simulink model "Basics_01"  (R2018a)
settings: Solver=VariableStepAuto  StartTime=0.0  StopTime=Ttot  RelTol=1e-3
values from neighbouring files (symbols this model uses):
  EnableInverter = 1    [Basics_00_Param.m]
  fn = 50    [Basics_00_Param.m]
  idref = 0.0    (= 0)    [Basics_00_Param.m]
  iqref_FinalLevel = -0.2    [Basics_00_Param.m]
  iqref_InitialLevel = 0.0    (= 0)    [Basics_00_Param.m]
  iqref_StepTime = 10000.760    (= 10000.76)    [Basics_00_Param.m]
  Kp = 2    [Basics_00_Param.m]
  L = X / 2 / pi / fn    (= 0.00159154943092)    [Basics_00_Param.m]
  Phi = atan (X/R)    [Basics_00_Param.m]
  R = X/20    (= 0.025)    [Basics_00_Param.m]
  Tau = L / R    (= 0.0636619772368)    [Basics_00_Param.m]
  Ts_control = 1/20000    (= 5e-05)    [Basics_00_Param.m]
  Ts_PWM = 1/200000    (= 5e-06)    [Basics_00_Param.m]
  Udc = Uanp * 3^0.5    (= 1.73205080757)    [Basics_00_Param.m]
  V_NegSeq_FinalValue = 0    [Basics_00_Param.m]
  V_NegSeq_InitialValue = 0.0    (= 0)    [Basics_00_Param.m]
  V_NegSeq_StepTime = 10000.25    [Basics_00_Param.m]
  V_PosSeq_FinalValue = 1    [Basics_00_Param.m]
  V_PosSeq_InitialValue = 1    [Basics_00_Param.m]
  V_PosSeq_StepTime = 10000    [Basics_00_Param.m]
  X = 0.5    [Basics_00_Param.m]
  Z = (X^2 + R^2)^0.5    (= 0.500624609863)    [Basics_00_Param.m]
undefined symbols (not defined in the file or in its folder): DDLPF_Notch, ESS, PCC, Select_AMA
libraries: PhD_Library x18, powerlib x10
settings Model: SimulationMode=accelerator  Creator=daniemot  LastModifiedBy=daniemot
settings SolverCC: AutoInsertRateTranBlk=on
settings DataIOCC: ExternalInput=getinputstruct(WN_50mF_op_snapshot1)  InitialState=getstatestruct(WN_50mF_op_snapshot1)  SaveFinalState=on  SaveFormat=StructureWithTime  SaveOutput=off  SignalLogging=off  DSMLogging=off  SaveTime=off
settings DebuggingCC: ReadBeforeWriteMsg=DisableAll  WriteAfterWriteMsg=DisableAll  WriteAfterReadMsg=DisableAll  MultiTaskDSMMsg=none
settings ModelReferenceCC: UpdateModelReferenceTargets=IfOutOfDate
settings SFSimCC: SFSimEcho=off

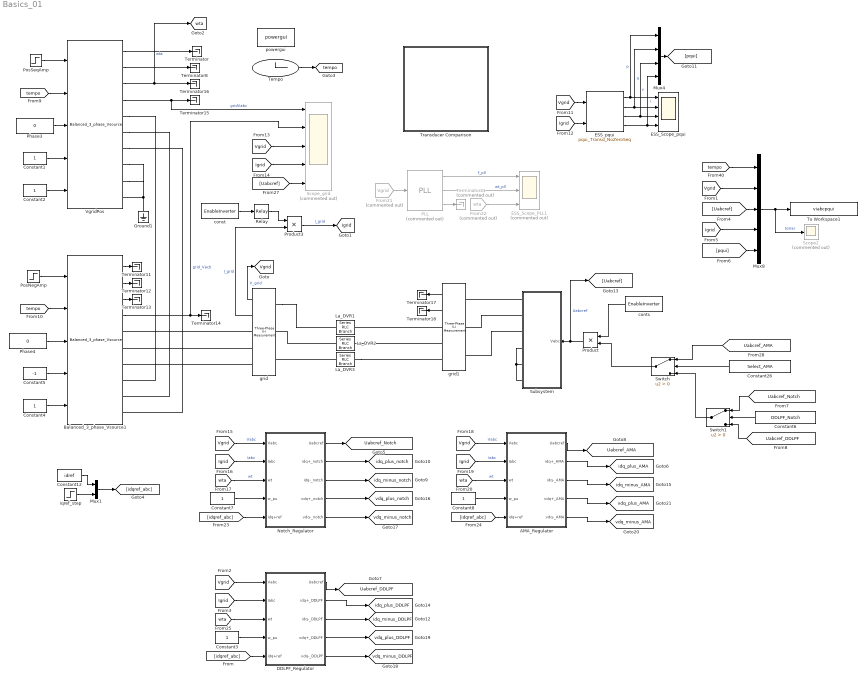
== system Basics_01 ==
  AMA_Regulator : Subsystem
  Balanced_3_phase_Vsource1 : PhD_Library/Offshore_Oil_and_Wind/Balanced_3_phase_Vsource  BaseAmp=Uanp  fn=fn
  Constant{1..4,7..8} (6 alike) : Constant
  Constant12 : Constant  Value=idref
  Constant26 : Constant  Value=Select_AMA
  Constant5 : Constant  Value=-1
  Constant6 : Constant  Value=DDLPF_Notch
  DDLPF_Regulator : Subsystem
  ESS_Scope_PLL1 : Scope  Commented=on  NumInputPorts=3
  ESS_Scope_pqui : Scope  NumInputPorts=4
  ESS_pqui : PhD_Library/Offshore_Oil_and_Wind/pqui_Transd_NoZeroSeq  Sn=3/2  Uanp=1  Iap=1
  From21 : From  Commented=on  GotoTag=Vgrid
  From22 : From  Commented=on  GotoTag=wta
  Ground1 : powerlib/Elements/Ground  LConnTagsString=a
  La_DVR1 : powerlib/Elements/Series RLC Branch  LConnTagsString=__new0  RConnTagsString=__new0  BranchType=RL  Resistance=R  Inductance=L  SetiL0=off  InitialCurrent=0  Capacitance=1.0  Setx0=off  InitialVoltage=0  Measurements=None
  La_DVR2 : powerlib/Elements/Series RLC Branch  LConnTagsString=__new0  RConnTagsString=__new0  BranchType=RL  Resistance=R  Inductance=L  SetiL0=off  InitialCurrent=0  Capacitance=1.0  Setx0=off  InitialVoltage=0  Measurements=None
  La_DVR3 : powerlib/Elements/Series RLC Branch  LConnTagsString=__new0  RConnTagsString=__new0  BranchType=RL  Resistance=R  Inductance=L  SetiL0=off  InitialCurrent=0  Capacitance=1.0  Setx0=off  InitialVoltage=0  Measurements=None
  Mux1 : Mux  Inputs=2
  Mux4 : Mux
  Mux8 : Mux  Inputs=5
  Notch_Regulator : Subsystem
  PLL : PhD_Library/Offshore_Oil_and_Wind/PLL  Commented=on  fn=fn  Ts=Ts_control  Kp_pll=90  Ki_pll=1600  Kd_pll=0  PLL_ini=0
  Phase3 : Constant  Value=0
  Phase4 : Constant  Value=0
  PosNegAmp : Step  Time=V_NegSeq_StepTime  Before=V_NegSeq_InitialValue  After=V_NegSeq_FinalValue
  PosSeqAmp : Step  Time=V_PosSeq_StepTime  Before=V_PosSeq_InitialValue  After=V_PosSeq_FinalValue
  Product : Product
  Product3 : Product
  Relay : Relay  OnSwitchValue=0.5  OffSwitchValue=0.4  OffOutputValue=-1
  Scope2 : Scope  Commented=on
  Scope_grid : Scope  Commented=on  NumInputPorts=5
  Subsystem : Subsystem
  Switch : Switch  Criteria=u2 > Threshold
  Switch1 : Switch  Criteria=u2 > Threshold
  Tempo : Clock
  Terminator{,8,11..18} (10 alike) : Terminator
  Terminator21 : Terminator  Commented=on
  To Workspace1 : ToWorkspace  VariableName=viabcpqui  SampleTime=Ts_control
  Transducer Comparison : Subsystem
  VgridPos : PhD_Library/Offshore_Oil_and_Wind/Balanced_3_phase_Vsource  BaseAmp=Uanp  fn=fn
  const : Constant  Value=EnableInverter
  conts : Constant  Value=EnableInverter
  grid : powerlib/Measurements/Three-Phase V-I Measurement  VoltageMeasurement=phase-to-ground  SetLabelV=off  LabelV=vconv  Vpu=off  VpuLL=off  CurrentMeasurement=yes  SetLabelI=off  LabelI=iconv  Ipu=off  Pbase=sn  Vbase=uab  OutputType=Complex  PhasorSimulation=off  PSBequivalent=0
  grid1 : powerlib/Measurements/Three-Phase V-I Measurement  VoltageMeasurement=phase-to-ground  SetLabelV=off  LabelV=vconv  Vpu=off  VpuLL=off  CurrentMeasurement=yes  SetLabelI=off  LabelI=iconv  Ipu=off  Pbase=sn  Vbase=uab  OutputType=Complex  PhasorSimulation=off  PSBequivalent=0
  iqref_step : Step  Time=iqref_StepTime  Before=iqref_InitialLevel  After=iqref_FinalLevel
  powergui : powerlib/powergui  Priority=1  SimulationMode=Discrete  SampleTime=5e-6  frequency=60  Iterations=50  frequencyindice=0  Pbase=100e6  ErrMax=1e-4  UnitsV=kV  UnitsW=MW  buscounter=0  FunctionMessages=off  echomessages=off  EnableUseOfTLC=off  CurrentSourceSwitches=off  DisableSnubberDevices=off  DisableRonSwitches=off  DisableVfSwitches=off  DisplayEquations=off  SolverType=Tustin/Backward Euler (TBE)  Interpol=off  ExternalGateDelay=off  methode=off  Ts=100  x0status=blocks  SPID=off  SwTol=0  HookPort=off  RestoreLinks=warning  ResistiveCurrentMeasurement=off  Frange=[0:2:500]  Ylog=off  Xlog=on  ShowGrid=off  save=off  variable=ZData  structure=0  ZoomFFT=off  StartTime=0.0  cycles=1  DisplayStyle=1  fundamental=60  FreqAxis=off  MaxFrequency=1000  frequencyindicesteady=1  RmsSteady=1  display=off
  tag scope: Igrid=global, Uabcref_AMA=global, Uabcref_DDLPF=global, Uabcref_Notch=global, Vgrid=global, idq_minus_AMA=global, idq_minus_DDLPF=global, idq_minus_notch=global, idq_plus_AMA=global, idq_plus_DDLPF=global, idq_plus_notch=global, tempo=global, vdq_minus_AMA=global, vdq_minus_DDLPF=global, vdq_minus_notch=global, vdq_plus_AMA=global, vdq_plus_DDLPF=global, vdq_plus_notch=global, wta=global
  wires:
  ESS_pqui/3 -> Mux4/3, ESS_Scope_pqui/3  "v"
  ESS_pqui/2 -> Mux4/2, ESS_Scope_pqui/2  "q"
  ESS_pqui/4 -> Mux4/4, ESS_Scope_pqui/4  "i"
  ESS_pqui/1 -> Mux4/1, ESS_Scope_pqui/1  "p"
  grid/1 -> [Vgrid]  "V_grid"
  Product3/1 -> [Igrid]  "I_grid"
  VgridPos/3 -> [wta], Terminator16/1  "wta"
  Constant1/1 -> VgridPos/4
  Constant2/1 -> VgridPos/5
  Tempo/1 -> [tempo]
  [tempo] -> VgridPos/2
  VgridPos/1 -> Terminator/1
  VgridPos/2 -> Terminator8/1
  PosSeqAmp/1 -> VgridPos/1
  Phase3/1 -> VgridPos/3
  PosNegAmp/1 -> Balanced_3_phase_Vsource1/1
  Phase4/1 -> Balanced_3_phase_Vsource1/3
  [tempo] -> Balanced_3_phase_Vsource1/2
  Constant4/1 -> Balanced_3_phase_Vsource1/5
  Constant5/1 -> Balanced_3_phase_Vsource1/4
  Balanced_3_phase_Vsource1/1 -> Terminator11/1
  Balanced_3_phase_Vsource1/2 -> Terminator12/1
  Balanced_3_phase_Vsource1/3 -> Terminator13/1
  Balanced_3_phase_Vsource1/4 -> Scope_grid/2, Terminator14/1  "grid_Vacb"
  VgridPos/4 -> Scope_grid/1, Terminator15/1  "gridVabc"
  grid1/1 -> Terminator17/1
  grid1/2 -> Terminator18/1
  [Vgrid] -> ESS_pqui/1
  [Igrid] -> ESS_pqui/2
  [Vgrid] -> Scope_grid/3
  [Igrid] -> Scope_grid/4
  From21/1 -> PLL/1
  PLL/1 -> ESS_Scope_PLL1/1  "f_pll"
  PLL/2 -> ESS_Scope_PLL1/2  "wt_pll"
  From22/1 -> ESS_Scope_PLL1/3
  PLL/3 -> Terminator21/1
  Mux1/1 -> [idqref_abc]
  iqref_step/1 -> Mux1/2
  Constant12/1 -> Mux1/1
  [Uabcref] -> Scope_grid/5
  Switch/1 -> Product/2
  [Uabcref_AMA] -> Switch/1
  Switch1/1 -> Switch/3
  Constant26/1 -> Switch/2
  Product/1 -> [Uabcref], Subsystem/1(Vabc)  "Uabcref"
  conts/1 -> Product/1
  grid/2 -> Product3/2  "I_grid"
  Relay/1 -> Product3/1
  const/1 -> Relay/1
  Mux8/1 -> Scope2/1, To Workspace1/1  "toVar"
  [tempo] -> Mux8/1
  [Vgrid] -> Mux8/2
  [Uabcref] -> Mux8/3
  [Igrid] -> Mux8/4
  Mux4/1 -> [pqui]
  [pqui] -> Mux8/5
  [Vgrid] -> DDLPF_Regulator/1(Vabc)
  [wta] -> DDLPF_Regulator/3(wt)
  [Igrid] -> DDLPF_Regulator/2(Iabc)
  DDLPF_Regulator/3(idq-_DDLPF) -> [idq_minus_DDLPF]
  DDLPF_Regulator/2(idq+_DDLPF) -> [idq_plus_DDLPF]
  DDLPF_Regulator/1(Uabcref) -> [Uabcref_DDLPF]
  [idqref_abc] -> DDLPF_Regulator/5(idq+ref)
  Constant3/1 -> DDLPF_Regulator/4(w_pu)
  [Vgrid] -> Notch_Regulator/1(Vabc)  "Vabc"
  [Igrid] -> Notch_Regulator/2(Iabc)  "Iabc"
  [wta] -> Notch_Regulator/3(wt)  "wt"
  Constant7/1 -> Notch_Regulator/4(w_pu)
  Notch_Regulator/1(Uabcref) -> [Uabcref_Notch]
  Notch_Regulator/2(idq+_notch) -> [idq_plus_notch]
  Notch_Regulator/3(idq-_notch) -> [idq_minus_notch]
  [Uabcref_Notch] -> Switch1/1
  Constant6/1 -> Switch1/2
  [Uabcref_DDLPF] -> Switch1/3
  AMA_Regulator/3(idq-_AMA) -> [idq_minus_AMA]
  AMA_Regulator/2(idq+_AMA) -> [idq_plus_AMA]
  [wta] -> AMA_Regulator/3(wt)  "wt"
  AMA_Regulator/1(Uabcref) -> [Uabcref_AMA]
  [Igrid] -> AMA_Regulator/2(Iabc)  "Iabc"
  [Vgrid] -> AMA_Regulator/1(Vabc)  "Vabc"
  Constant8/1 -> AMA_Regulator/4(w_pu)
  [idqref_abc] -> Notch_Regulator/5(idq+ref)
  [idqref_abc] -> AMA_Regulator/5(idq+ref)
  Notch_Regulator/5(vdq-_notch) -> [vdq_minus_notch]
  Notch_Regulator/4(vdq+_notch) -> [vdq_plus_notch]
  DDLPF_Regulator/4(vdq+_DDLPF) -> [vdq_plus_DDLPF]
  DDLPF_Regulator/5(vdq-_DDLPF) -> [vdq_minus_DDLPF]
  AMA_Regulator/4(vdq+_AMA) -> [vdq_plus_AMA]
  AMA_Regulator/5(vdq-_AMA) -> [vdq_minus_AMA]
  connections:
  Ground1/LConn1 -- VgridPos/RConn4 -- VgridPos/RConn5 -- VgridPos/RConn6
  VgridPos/RConn1 -- Balanced_3_phase_Vsource1/RConn4
  VgridPos/RConn2 -- Balanced_3_phase_Vsource1/RConn5
  VgridPos/RConn3 -- Balanced_3_phase_Vsource1/RConn6
  grid/LConn1 -- La_DVR1/RConn1
  La_DVR2/RConn1 -- grid/LConn2
  La_DVR3/RConn1 -- grid/LConn3
  grid/RConn1 -- Balanced_3_phase_Vsource1/RConn1
  grid/RConn2 -- Balanced_3_phase_Vsource1/RConn2
  grid/RConn3 -- Balanced_3_phase_Vsource1/RConn3
  grid1/RConn1 -- La_DVR1/LConn1
  La_DVR2/LConn1 -- grid1/RConn2
  La_DVR3/LConn1 -- grid1/RConn3
  Subsystem/RConn4 -- Subsystem/RConn6 -- Subsystem/RConn5
  Subsystem/RConn1 -- grid1/LConn1
  Subsystem/RConn2 -- grid1/LConn2
  Subsystem/RConn3 -- grid1/LConn3

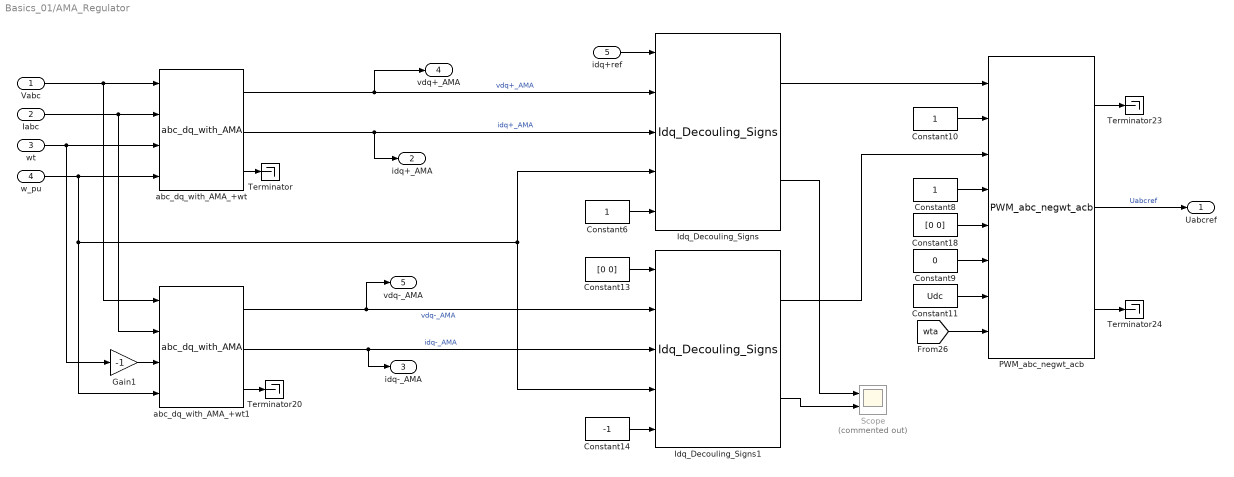
== system Basics_01/AMA_Regulator ==
  Vabc : Inport
  Iabc : Inport  Port=2
  wt : Inport  Port=3
  w_pu : Inport  Port=4
  idq+ref : Inport  Port=5
  Constant10 : Constant
  Constant11 : Constant  Value=Udc
  Constant13 : Constant  Value=[0 0]
  Constant14 : Constant  Value=-1
  Constant18 : Constant  Value=[0 0]
  Constant6 : Constant
  Constant8 : Constant
  Constant9 : Constant  Value=0
  Gain1 : Gain  Gain=-1
  Idq_Decouling_Signs : PhD_Library/Offshore_Oil_and_Wind/Idq_Decouling_Signs  Ts=Ts_control  fn=fn  Kp=Kp  Ti=Ti  I_ini_d=0  I_ini_q=0  L=X  PI_max=1.5  PI_min=-1.5  TrafoPhaseComp=0
  Idq_Decouling_Signs1 : PhD_Library/Offshore_Oil_and_Wind/Idq_Decouling_Signs  Ts=Ts_control  fn=fn  Kp=Kp  Ti=Ti  I_ini_d=0  I_ini_q=0  L=X  PI_max=1.5  PI_min=-1.5  TrafoPhaseComp=0
  PWM_abc_negwt_acb : PhD_Library/Offshore_Oil_and_Wind/PWM_abc_negwt_acb  fsw=fsw  Ts=Ts_PWM  Uabp=Uabp  PWM_Ini_Phase=90
  Scope : Scope  Commented=on  NumInputPorts=2
  Terminator{,20,23..24} (4 alike) : Terminator
  abc_dq_with_AMA_+wt : PhD_Library/Offshore_Oil_and_Wind/abc_dq_with_AMA  Ts=Ts_control  fn=fn  fmin=fn*0.8  fmax=fn*1.2  fcutoutv=f_LPF_noise  fcutouti=f_LPF_noise
  abc_dq_with_AMA_+wt1 : PhD_Library/Offshore_Oil_and_Wind/abc_dq_with_AMA  Ts=Ts_control  fn=fn  fmin=fn*0.8  fmax=fn*1.2  fcutoutv=f_LPF_noise  fcutouti=f_LPF_noise
  Uabcref : Outport
  idq+_AMA : Outport  Port=2
  idq-_AMA : Outport  Port=3
  vdq+_AMA : Outport  Port=4
  vdq-_AMA : Outport  Port=5
  wires:
  Constant18/1 -> PWM_abc_negwt_acb/5
  Constant11/1 -> PWM_abc_negwt_acb/7
  abc_dq_with_AMA_+wt1/1 -> vdq-_AMA/1, Idq_Decouling_Signs1/2  "vdq-_AMA"
  wt/1 -> abc_dq_with_AMA_+wt/3, Gain1/1
  PWM_abc_negwt_acb/3 -> Terminator24/1
  Constant13/1 -> Idq_Decouling_Signs1/1
  Gain1/1 -> abc_dq_with_AMA_+wt1/3
  Constant14/1 -> Idq_Decouling_Signs1/5
  abc_dq_with_AMA_+wt1/3 -> Terminator20/1
  Idq_Decouling_Signs/2 -> Scope/1
  abc_dq_with_AMA_+wt/1 -> vdq+_AMA/1, Idq_Decouling_Signs/2  "vdq+_AMA"
  Idq_Decouling_Signs1/1 -> PWM_abc_negwt_acb/3
  abc_dq_with_AMA_+wt1/2 -> idq-_AMA/1, Idq_Decouling_Signs1/3  "idq-_AMA"
  Constant10/1 -> PWM_abc_negwt_acb/2
  idq+ref/1 -> Idq_Decouling_Signs/1
  Constant8/1 -> PWM_abc_negwt_acb/4
  Constant6/1 -> Idq_Decouling_Signs/5
  [wta] -> PWM_abc_negwt_acb/8
  abc_dq_with_AMA_+wt/2 -> idq+_AMA/1, Idq_Decouling_Signs/3  "idq+_AMA"
  Constant9/1 -> PWM_abc_negwt_acb/6
  Idq_Decouling_Signs/1 -> PWM_abc_negwt_acb/1
  PWM_abc_negwt_acb/1 -> Terminator23/1
  PWM_abc_negwt_acb/2 -> Uabcref/1  "Uabcref"
  Iabc/1 -> abc_dq_with_AMA_+wt1/2, abc_dq_with_AMA_+wt/2
  abc_dq_with_AMA_+wt/3 -> Terminator/1
  w_pu/1 -> abc_dq_with_AMA_+wt1/4, Idq_Decouling_Signs/4, Idq_Decouling_Signs1/4, abc_dq_with_AMA_+wt/4
  Vabc/1 -> abc_dq_with_AMA_+wt1/1, abc_dq_with_AMA_+wt/1
  Idq_Decouling_Signs1/2 -> Scope/2

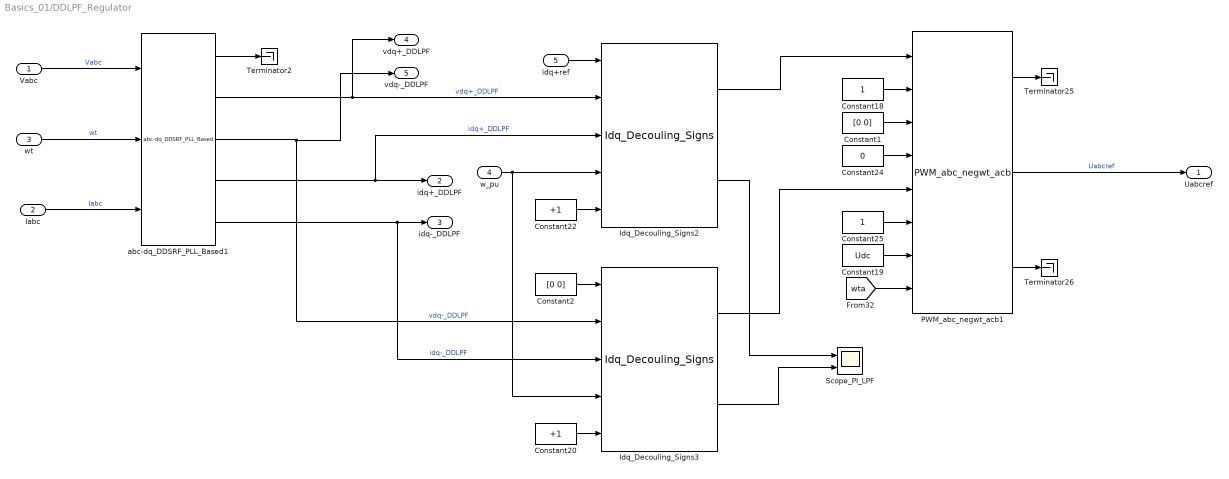
== system Basics_01/DDLPF_Regulator ==
  Vabc : Inport
  Iabc : Inport  Port=2
  wt : Inport  Port=3
  w_pu : Inport  Port=4
  idq+ref : Inport  Port=5
  Constant1 : Constant  Value=[0 0]
  Constant18 : Constant
  Constant19 : Constant  Value=Udc
  Constant2 : Constant  Value=[0 0]
  Constant20 : Constant  Value=+1
  Constant22 : Constant  Value=+1
  Constant24 : Constant  Value=0
  Constant25 : Constant
  Idq_Decouling_Signs2 : PhD_Library/Offshore_Oil_and_Wind/Idq_Decouling_Signs  Ts=Ts_control  fn=fn  Kp=Kp  Ti=Ti  I_ini_d=0  I_ini_q=0  L=X  PI_max=1.5  PI_min=-1.5  TrafoPhaseComp=0
  Idq_Decouling_Signs3 : PhD_Library/Offshore_Oil_and_Wind/Idq_Decouling_Signs  Ts=Ts_control  fn=fn  Kp=Kp  Ti=Ti  I_ini_d=0  I_ini_q=0  L=X  PI_max=1.5  PI_min=-1.5  TrafoPhaseComp=0
  PWM_abc_negwt_acb1 : PhD_Library/Offshore_Oil_and_Wind/PWM_abc_negwt_acb  fsw=fsw  Ts=Ts_PWM  Uabp=Uabp  PWM_Ini_Phase=90
  Scope_PI_LPF : Scope  NumInputPorts=2
  Terminator2 : Terminator
  Terminator25 : Terminator
  Terminator26 : Terminator
  abc-dq_DDSRF_PLL_Based1 : PhD_Library/Offshore_Oil_and_Wind/abc-dq_DDSRF_PLL_Based  Ts=Ts_control  fc=fn/2^0.5
  Uabcref : Outport
  idq+_DDLPF : Outport  Port=2
  idq-_DDLPF : Outport  Port=3
  vdq+_DDLPF : Outport  Port=4
  vdq-_DDLPF : Outport  Port=5
  wires:
  Constant19/1 -> PWM_abc_negwt_acb1/7
  w_pu/1 -> Idq_Decouling_Signs3/4, Idq_Decouling_Signs2/4
  abc-dq_DDSRF_PLL_Based1/4 -> idq+_DDLPF/1, Idq_Decouling_Signs2/3  "idq+_DDLPF"
  abc-dq_DDSRF_PLL_Based1/2 -> vdq+_DDLPF/1, Idq_Decouling_Signs2/2  "vdq+_DDLPF"
  idq+ref/1 -> Idq_Decouling_Signs2/1
  Idq_Decouling_Signs2/1 -> PWM_abc_negwt_acb1/1
  PWM_abc_negwt_acb1/1 -> Terminator25/1
  PWM_abc_negwt_acb1/3 -> Terminator26/1
  Constant24/1 -> PWM_abc_negwt_acb1/4
  Constant25/1 -> PWM_abc_negwt_acb1/6
  abc-dq_DDSRF_PLL_Based1/5 -> idq-_DDLPF/1, Idq_Decouling_Signs3/3  "idq-_DDLPF"
  abc-dq_DDSRF_PLL_Based1/3 -> vdq-_DDLPF/1, Idq_Decouling_Signs3/2  "vdq-_DDLPF"
  Idq_Decouling_Signs3/1 -> PWM_abc_negwt_acb1/5
  wt/1 -> abc-dq_DDSRF_PLL_Based1/2  "wt"
  Constant2/1 -> Idq_Decouling_Signs3/1
  Constant22/1 -> Idq_Decouling_Signs2/5
  Constant18/1 -> PWM_abc_negwt_acb1/2
  Idq_Decouling_Signs2/2 -> Scope_PI_LPF/1
  [wta] -> PWM_abc_negwt_acb1/8
  Constant1/1 -> PWM_abc_negwt_acb1/3
  Constant20/1 -> Idq_Decouling_Signs3/5
  abc-dq_DDSRF_PLL_Based1/1 -> Terminator2/1
  Vabc/1 -> abc-dq_DDSRF_PLL_Based1/1  "Vabc"
  Iabc/1 -> abc-dq_DDSRF_PLL_Based1/3  "Iabc"
  PWM_abc_negwt_acb1/2 -> Uabcref/1  "Uabcref"
  Idq_Decouling_Signs3/2 -> Scope_PI_LPF/2

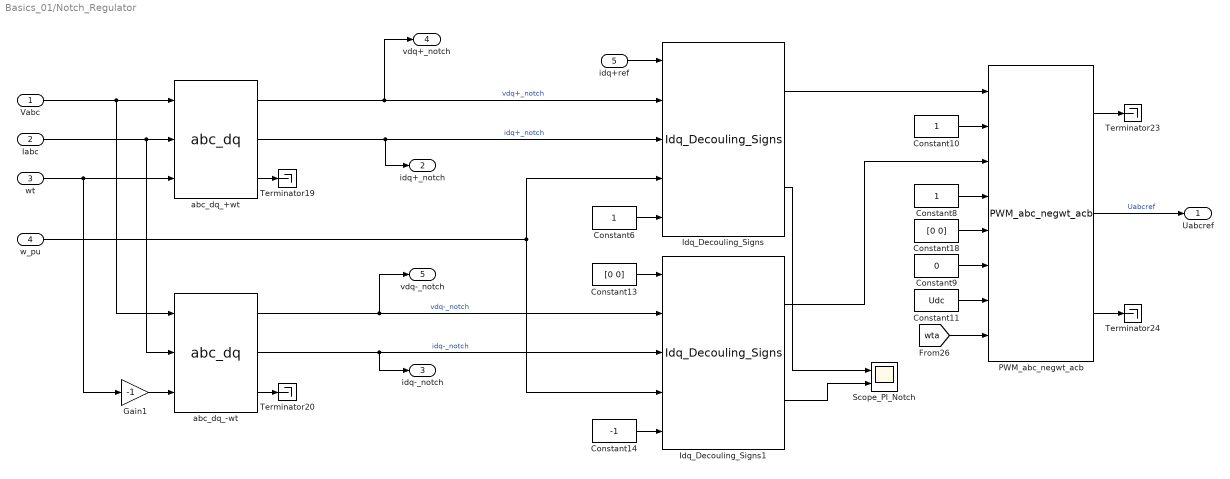
== system Basics_01/Notch_Regulator ==
  Vabc : Inport
  Iabc : Inport  Port=2
  wt : Inport  Port=3
  w_pu : Inport  Port=4
  idq+ref : Inport  Port=5
  Constant10 : Constant
  Constant11 : Constant  Value=Udc
  Constant13 : Constant  Value=[0 0]
  Constant14 : Constant  Value=-1
  Constant18 : Constant  Value=[0 0]
  Constant6 : Constant
  Constant8 : Constant
  Constant9 : Constant  Value=0
  Gain1 : Gain  Gain=-1
  Idq_Decouling_Signs : PhD_Library/Offshore_Oil_and_Wind/Idq_Decouling_Signs  Ts=Ts_control  fn=fn  Kp=Kp  Ti=Ti  I_ini_d=0  I_ini_q=0  L=X  PI_max=1.5  PI_min=-1.5  TrafoPhaseComp=0
  Idq_Decouling_Signs1 : PhD_Library/Offshore_Oil_and_Wind/Idq_Decouling_Signs  Ts=Ts_control  fn=fn  Kp=Kp  Ti=Ti  I_ini_d=0  I_ini_q=0  L=X  PI_max=1.5  PI_min=-1.5  TrafoPhaseComp=0
  PWM_abc_negwt_acb : PhD_Library/Offshore_Oil_and_Wind/PWM_abc_negwt_acb  fsw=fsw  Ts=Ts_PWM  Uabp=Uabp  PWM_Ini_Phase=90
  Scope_PI_Notch : Scope  NumInputPorts=2
  Terminator{19..20,23..24} (4 alike) : Terminator
  abc_dq_+wt : PhD_Library/Offshore_Oil_and_Wind/abc_dq  Ts=Ts_control  fn=2*fn  fcutoutv=f_LPF_noise  fcutouti=f_LPF_noise  zeta=zeta
      link override Second-Order Filter2: PlotResponse=off
  abc_dq_-wt : PhD_Library/Offshore_Oil_and_Wind/abc_dq  Ts=Ts_control  fn=2*fn  fcutoutv=f_LPF_noise  fcutouti=f_LPF_noise  zeta=zeta
  Uabcref : Outport
  idq+_notch : Outport  Port=2
  idq-_notch : Outport  Port=3
  vdq+_notch : Outport  Port=4
  vdq-_notch : Outport  Port=5
  wires:
  Vabc/1 -> abc_dq_-wt/1, abc_dq_+wt/1
  Constant18/1 -> PWM_abc_negwt_acb/5
  Constant11/1 -> PWM_abc_negwt_acb/7
  abc_dq_-wt/1 -> vdq-_notch/1, Idq_Decouling_Signs1/2  "vdq-_notch"
  w_pu/1 -> Idq_Decouling_Signs/4, Idq_Decouling_Signs1/4
  wt/1 -> Gain1/1, abc_dq_+wt/3
  PWM_abc_negwt_acb/3 -> Terminator24/1
  Constant13/1 -> Idq_Decouling_Signs1/1
  Gain1/1 -> abc_dq_-wt/3
  Constant14/1 -> Idq_Decouling_Signs1/5
  abc_dq_-wt/3 -> Terminator20/1
  Idq_Decouling_Signs/2 -> Scope_PI_Notch/1
  abc_dq_+wt/1 -> vdq+_notch/1, Idq_Decouling_Signs/2  "vdq+_notch"
  Idq_Decouling_Signs1/1 -> PWM_abc_negwt_acb/3
  abc_dq_-wt/2 -> idq-_notch/1, Idq_Decouling_Signs1/3  "idq-_notch"
  Constant10/1 -> PWM_abc_negwt_acb/2
  idq+ref/1 -> Idq_Decouling_Signs/1
  Constant8/1 -> PWM_abc_negwt_acb/4
  Constant6/1 -> Idq_Decouling_Signs/5
  [wta] -> PWM_abc_negwt_acb/8
  abc_dq_+wt/2 -> idq+_notch/1, Idq_Decouling_Signs/3  "idq+_notch"
  Constant9/1 -> PWM_abc_negwt_acb/6
  Idq_Decouling_Signs/1 -> PWM_abc_negwt_acb/1
  PWM_abc_negwt_acb/1 -> Terminator23/1
  abc_dq_+wt/3 -> Terminator19/1
  Iabc/1 -> abc_dq_-wt/2, abc_dq_+wt/2
  PWM_abc_negwt_acb/2 -> Uabcref/1  "Uabcref"
  Idq_Decouling_Signs1/2 -> Scope_PI_Notch/2

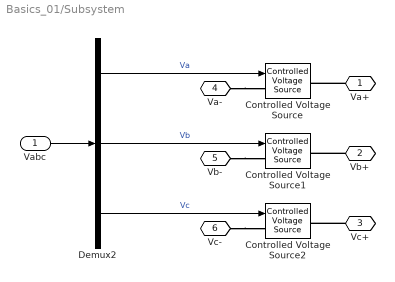
== system Basics_01/Subsystem ==
  Vabc : Inport
  Controlled Voltage Source : powerlib/Electrical Sources/Controlled Voltage Source  Initialize=off  Source_Type=AC  Amplitude=ESS.LSC.Ub*(2/3)^0.5  Phase=0  Frequency=PCC.fn  Measurements=None
  Controlled Voltage Source1 : powerlib/Electrical Sources/Controlled Voltage Source  Initialize=off  Source_Type=AC  Amplitude=ESS.LSC.Ub*(2/3)^0.5  Phase=-120  Frequency=PCC.fn  Measurements=None
  Controlled Voltage Source2 : powerlib/Electrical Sources/Controlled Voltage Source  Initialize=off  Source_Type=AC  Amplitude=ESS.LSC.Ub*(2/3)^0.5  Phase=120  Frequency=PCC.fn  Measurements=None
  Demux2 : Demux  Outputs=3
  Va+ : PMIOPort  Side=Right
  Vb+ : PMIOPort  Port=2  Side=Right
  Vc+ : PMIOPort  Port=3  Side=Right
  Va- : PMIOPort  Port=4  Side=Right
  Vb- : PMIOPort  Port=5  Side=Right
  Vc- : PMIOPort  Port=6  Side=Right
  wires:
  Demux2/1 -> Controlled Voltage Source/1  "Va"
  Demux2/2 -> Controlled Voltage Source1/1  "Vb"
  Demux2/3 -> Controlled Voltage Source2/1  "Vc"
  Vabc/1 -> Demux2/1
  connections:
  Va-/RConn1 -- Controlled Voltage Source/LConn1
  Va+/RConn1 -- Controlled Voltage Source/RConn1
  Vb-/RConn1 -- Controlled Voltage Source1/LConn1
  Vc-/RConn1 -- Controlled Voltage Source2/LConn1
  Vb+/RConn1 -- Controlled Voltage Source1/RConn1
  Vc+/RConn1 -- Controlled Voltage Source2/RConn1

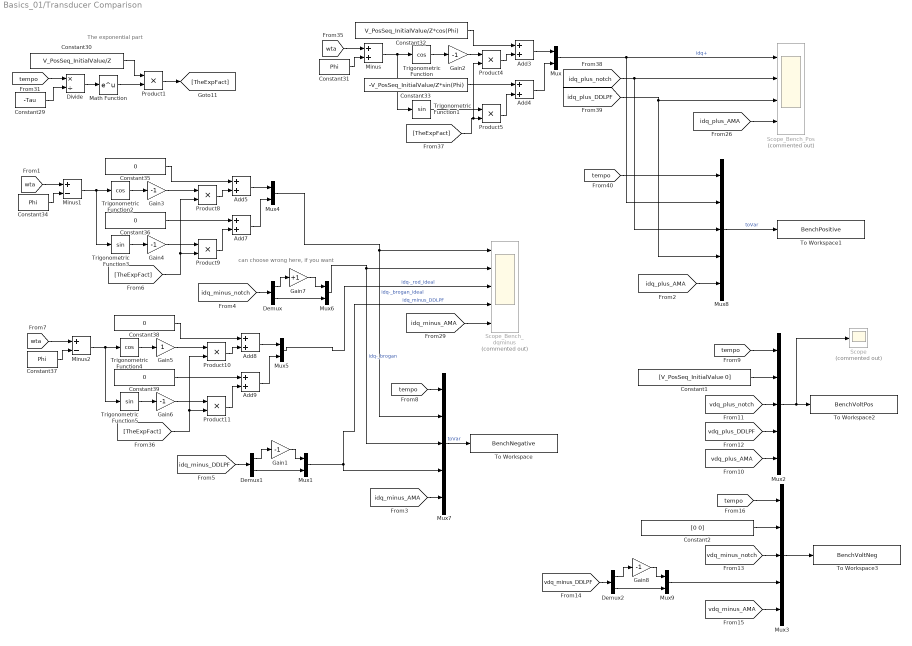
== system Basics_01/Transducer Comparison ==
  note: The exponential part
  note: can choose wrong here, if you want
  Add{3..5,7..9} (6 alike) : Sum
  Constant1 : Constant  Value=[V_PosSeq_InitialValue 0]
  Constant2 : Constant  Value=[0 0]
  Constant29 : Constant  Value=-Tau
  Constant30 : Constant  Value=V_PosSeq_InitialValue/Z
  Constant31 : Constant  Value=Phi
  Constant32 : Constant  Value=V_PosSeq_InitialValue/Z*cos(Phi)
  Constant33 : Constant  Value=-V_PosSeq_InitialValue/Z*sin(Phi)
  Constant34 : Constant  Value=Phi
  Constant{35..36,38..39} (4 alike) : Constant  Value=0
  Constant37 : Constant  Value=Phi
  Demux : Demux  Outputs=2
  Demux1 : Demux  Outputs=2
  Demux2 : Demux  Outputs=2
  Divide : Product  Inputs=*/
  Gain{1..4,6,8} (6 alike) : Gain  Gain=-1
  Gain5 : Gain
  Gain7 : Gain  Gain=+1
  Math Function : Math  SaturateOnIntegerOverflow=on
  Minus : Sum
  Minus1 : Sum  Inputs=+-
  Minus2 : Sum  Inputs=+-
  Mux{,1,4..6,9} (6 alike) : Mux  Inputs=2
  Mux{2..3,7..8} (4 alike) : Mux  Inputs=5
  Product{1,4..5,8..11} (7 alike) : Product
  Scope : Scope  Commented=on
  Scope_Bench_Pos : Scope  Commented=on  NumInputPorts=4
  Scope_Bench_dqminus : Scope  Commented=on  NumInputPorts=5
  To Workspace : ToWorkspace  VariableName=BenchNegative  SampleTime=Ts_control
  To Workspace1 : ToWorkspace  VariableName=BenchPositive  SampleTime=Ts_control
  To Workspace2 : ToWorkspace  VariableName=BenchVoltPos  SampleTime=Ts_control
  To Workspace3 : ToWorkspace  VariableName=BenchVoltNeg  SampleTime=Ts_control
  Trigonometric Function : Trigonometry  Operator=cos
  Trigonometric Function1 : Trigonometry
  Trigonometric Function2 : Trigonometry  Operator=cos
  Trigonometric Function3 : Trigonometry
  Trigonometric Function4 : Trigonometry  Operator=cos
  Trigonometric Function5 : Trigonometry
  wires:
  Add7/1 -> Mux4/2
  Constant35/1 -> Add5/1
  Product11/1 -> Add9/2
  Product1/1 -> [TheExpFact]
  Gain6/1 -> Product11/1
  Gain5/1 -> Product10/1
  Trigonometric Function4/1 -> Gain5/1
  [tempo] -> Mux7/1
  Trigonometric Function/1 -> Gain2/1
  [wta] -> Minus1/1
  Constant38/1 -> Add8/1
  Minus/1 -> Trigonometric Function1/1, Trigonometric Function/1
  Gain3/1 -> Product8/1
  Constant32/1 -> Add3/1
  Product9/1 -> Add7/2
  Divide/1 -> Math Function/1
  Add3/1 -> Mux/1
  Constant31/1 -> Minus/2
  Mux6/1 -> Mux7/3, Scope_Bench_dqminus/2  "idq-_brogan"
  Trigonometric Function5/1 -> Gain6/1
  Add5/1 -> Mux4/1
  [wta] -> Minus/1
  Mux8/1 -> To Workspace1/1  "toVar"
  Constant33/1 -> Add4/1
  [TheExpFact] -> Product8/2, Product9/2
  Constant34/1 -> Minus1/2
  [idq_minus_notch] -> Demux/1
  Product5/1 -> Add4/2
  Mux7/1 -> To Workspace/1  "toVar"
  Add8/1 -> Mux5/1
  Constant39/1 -> Add9/1
  Product8/1 -> Add5/2
  Constant29/1 -> Divide/2
  Trigonometric Function1/1 -> Product5/1
  Mux4/1 -> Mux7/2, Scope_Bench_dqminus/1  "idq-_brogan_ideal"
  Product10/1 -> Add8/2
  [tempo] -> Divide/1
  Gain2/1 -> Product4/1
  Gain4/1 -> Product9/1
  Minus2/1 -> Trigonometric Function5/1, Trigonometric Function4/1
  Mux5/1 -> Scope_Bench_dqminus/3  "idq-_rod_ideal"
  Add9/1 -> Mux5/2
  Mux/1 -> Mux8/2, Scope_Bench_Pos/1  "idq+"
  [TheExpFact] -> Product4/2, Product5/2
  [idq_plus_DDLPF] -> Mux8/4, Scope_Bench_Pos/3
  Demux/1 -> Gain7/1
  Mux1/1 -> Mux7/4, Scope_Bench_dqminus/4  "idq_minus_DDLPF"
  Constant37/1 -> Minus2/2
  Math Function/1 -> Product1/2
  Gain7/1 -> Mux6/1
  Add4/1 -> Mux/2
  Demux/2 -> Mux6/2
  [tempo] -> Mux8/1
  [idq_plus_notch] -> Mux8/3, Scope_Bench_Pos/2
  Constant30/1 -> Product1/1
  [TheExpFact] -> Product10/2, Product11/2
  [wta] -> Minus2/1
  Trigonometric Function2/1 -> Gain3/1
  Minus1/1 -> Trigonometric Function3/1, Trigonometric Function2/1
  Trigonometric Function3/1 -> Gain4/1
  Constant36/1 -> Add7/1
  Product4/1 -> Add3/2
  [idq_plus_AMA] -> Scope_Bench_Pos/4
  [idq_minus_AMA] -> Scope_Bench_dqminus/5
  Demux1/1 -> Gain1/1
  [idq_minus_DDLPF] -> Demux1/1
  Gain1/1 -> Mux1/1
  Demux1/2 -> Mux1/2
  [idq_plus_AMA] -> Mux8/5
  [idq_minus_AMA] -> Mux7/5
  [tempo] -> Mux2/1
  Constant1/1 -> Mux2/2
  Mux2/1 -> Scope/1, To Workspace2/1
  [vdq_plus_AMA] -> Mux2/5
  [vdq_plus_DDLPF] -> Mux2/4
  [vdq_plus_notch] -> Mux2/3
  [vdq_minus_AMA] -> Mux3/5
  Mux3/1 -> To Workspace3/1
  [vdq_minus_notch] -> Mux3/3
  [tempo] -> Mux3/1
  Constant2/1 -> Mux3/2
  Mux9/1 -> Mux3/4
  Demux2/1 -> Gain8/1
  Demux2/2 -> Mux9/2
  Gain8/1 -> Mux9/1
  [vdq_minus_DDLPF] -> Demux2/1
